simulink model "Lag_Optimal_Pole_Cancellation"  (R2022b)
settings: Solver=VariableStepAuto  StartTime=0.0  StopTime=15  RelTol=1e-3
undefined symbols (not defined in the file): k, p, p2, z2
libraries: simulink x3
settings Model: Creator=amirz  LastModifiedBy=amirz

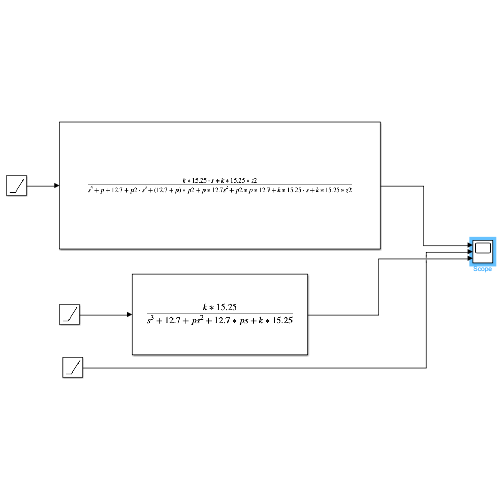
[thumbnail: Simulink's stored preview of the top-level diagram]
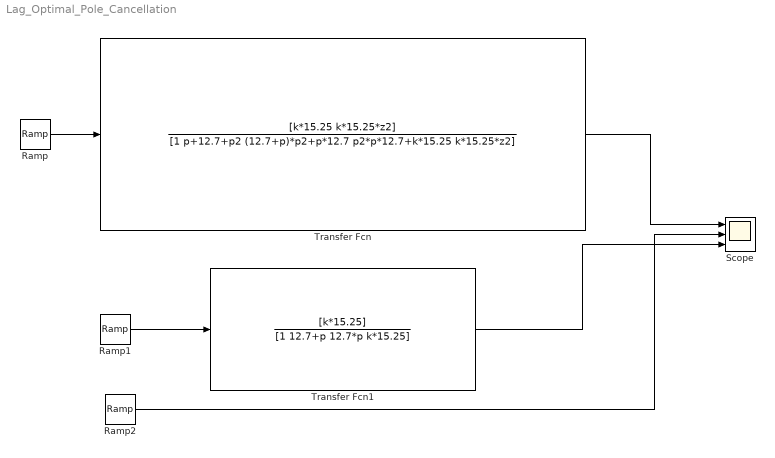
== system Lag_Optimal_Pole_Cancellation ==
  Ramp : simulink/Sources/Ramp  slope=1  start=0  InitialOutput=0
  Ramp1 : simulink/Sources/Ramp  slope=1  start=0  InitialOutput=0
  Ramp2 : simulink/Sources/Ramp  slope=1  start=0  InitialOutput=0
  Scope : Scope  NumInputPorts=3
  Transfer Fcn : TransferFcn  Numerator=[k*15.25 k*15.25*z2]  Denominator=[1 p+12.7+p2 (12.7+p)*p2+p*12.7 p2*p*12.7+k*15.25 k*15.25*z2]
  Transfer Fcn1 : TransferFcn  Numerator=[k*15.25]  Denominator=[1 12.7+p 12.7*p k*15.25]
  wires:
  Ramp1/1 -> Transfer Fcn1/1
  Ramp/1 -> Transfer Fcn/1
  Transfer Fcn/1 -> Scope/1
  Transfer Fcn1/1 -> Scope/3
  Ramp2/1 -> Scope/2
